simulink model "ADRClibriry"  (R2018a)
settings: Solver=VariableStepAuto  StartTime=0.0  StopTime=10.0  RelTol=1e-3
undefined symbols (not defined in the file or in its folder): sigbuilder_block
libraries: simulink x7, dspswit3 x4
(part 1 of 2)
settings Model: Creator=mengc  LastModifiedBy=mengc

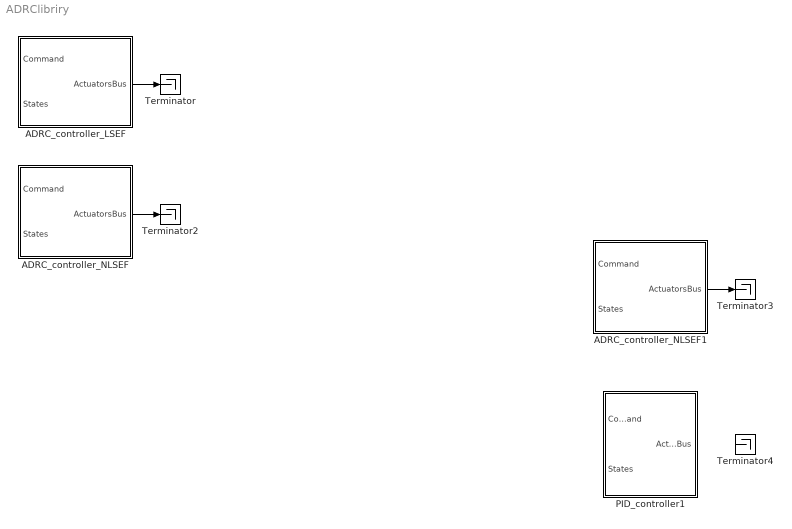
== system ADRClibriry ==
  ADRC_controller_LSEF : Subsystem
  ADRC_controller_NLSEF : Subsystem
  ADRC_controller_NLSEF1 : Subsystem
  PID_controller1 : Subsystem
  Terminator{,2..4} (4 alike) : Terminator
  wires:
  ? -> ADRC_controller_NLSEF/1(Command)  "Command"
  ADRC_controller_NLSEF/1(ActuatorsBus) -> Terminator2/1
  ? -> ADRC_controller_LSEF/1(Command)  "Command"
  ? -> ADRC_controller_LSEF/2(States)  "States"
  ? -> ADRC_controller_NLSEF/2(States)  "States"
  ADRC_controller_LSEF/1(ActuatorsBus) -> Terminator/1
  ? -> PID_controller1/1(Command)  "Command"
  ADRC_controller_NLSEF1/1(ActuatorsBus) -> Terminator3/1
  ? -> ADRC_controller_NLSEF1/2(States)  "States"
  ? -> ADRC_controller_NLSEF1/1(Command)  "Command"
  ? -> PID_controller1/2(States)  "States"

== system ADRClibriry/ADRC_controller_LSEF ==
  Command : Inport
  States : Inport  Port=2  OutDataTypeStr=Bus: StatesBus
  Bus Creator : BusCreator  Inputs=5  OutDataTypeStr=Bus: ActuatorsBus
  Bus Selector : BusSelector  OutputSignals=roll_cmd,pitch_cmd,yaw_cmd,throttle_cmd
  Bus Selector1 : BusSelector  OutputSignals=Omega_body,Euler
  Constant1 : Constant  Value=1225
  Demux : Demux  Outputs=3
  Demux1 : Demux  Outputs=3
  N-Sample Switch : dspswit3/N-Sample Switch  N=3  reset=off  TriggerType=Rising edge  Ts=0.01
      settings: SourceProductName=DSP System Toolbox  SourceProductBaseCode=DS
  Saturation : Saturate  UpperLimit=0  LowerLimit=-9.788*2
  Subsystem : Subsystem
  Subsystem2 : Subsystem
  Subsystem3 : Subsystem
  Terminator : Terminator
  Terminator1 : Terminator
  Unit Delay2 : UnitDelay  SampleTime=-1
  h_ADRC : Subsystem
  h_ADRC2 : Subsystem
  h_ADRC3 : Subsystem
  pitch_ADRC : Subsystem
  roll_ADRC : Subsystem
  yaw_ADRC : Subsystem
  ActuatorsBus : Outport  OutDataTypeStr=Bus: ActuatorsBus
  wires:
  Command/1 -> Bus Selector/1
  Unit Delay2/1 -> roll_ADRC/1(States), Bus Selector1/1, h_ADRC/1(States), yaw_ADRC/1(States), pitch_ADRC/1(States)
  yaw_ADRC/1(u_r) -> Subsystem3/3(u_r)
  Subsystem2/4(c4) -> Bus Creator/4
  Bus Selector1/2 -> Demux/1  "<Euler>"
  Bus Creator/1 -> ActuatorsBus/1  "ActuatorsBus"
  Bus Selector1/1 -> Demux1/1  "<Omega_body>"
  Demux/3 -> Terminator/1
  Subsystem3/2(u_2) -> Subsystem2/2(u_2)
  Subsystem3/1(u_1) -> Subsystem2/1(u_1)
  roll_ADRC/1("u_p ") -> Subsystem3/1(u_p)
  h_ADRC/1(a_t) -> Saturation/1
  Saturation/1 -> Subsystem/3(In3)
  Demux/1 -> Subsystem/1(In1)
  Demux/2 -> Subsystem/2(In2)
  Demux1/2 -> Subsystem3/5(q)
  Demux1/3 -> Terminator1/1
  N-Sample Switch/1 -> Bus Creator/5, Subsystem3/6(speed)  "speed"
  Constant1/1 -> N-Sample Switch/1
  Subsystem/1(speed) -> N-Sample Switch/2  "speed"
  Subsystem3/3(u_3) -> Subsystem2/3(u_3)
  Subsystem2/1(c1) -> Bus Creator/1
  Subsystem2/3(c3) -> Bus Creator/3
  Subsystem2/2(c2) -> Bus Creator/2
  pitch_ADRC/1(u_q) -> Subsystem3/2(u_q)
  Demux1/1 -> Subsystem3/4(p)
  Bus Selector/1 -> roll_ADRC/2(<roll_cmd>)  "<roll_cmd>"
  States/1 -> Unit Delay2/1
  Bus Selector/2 -> pitch_ADRC/2(<pitch_cmd>)  "<pitch_cmd>"
  Bus Selector/3 -> yaw_ADRC/2(<yaw_cmd>)  "<yaw_cmd>"
  Bus Selector/4 -> h_ADRC/2(<throttle_cmd>)  "<throttle_cmd>"

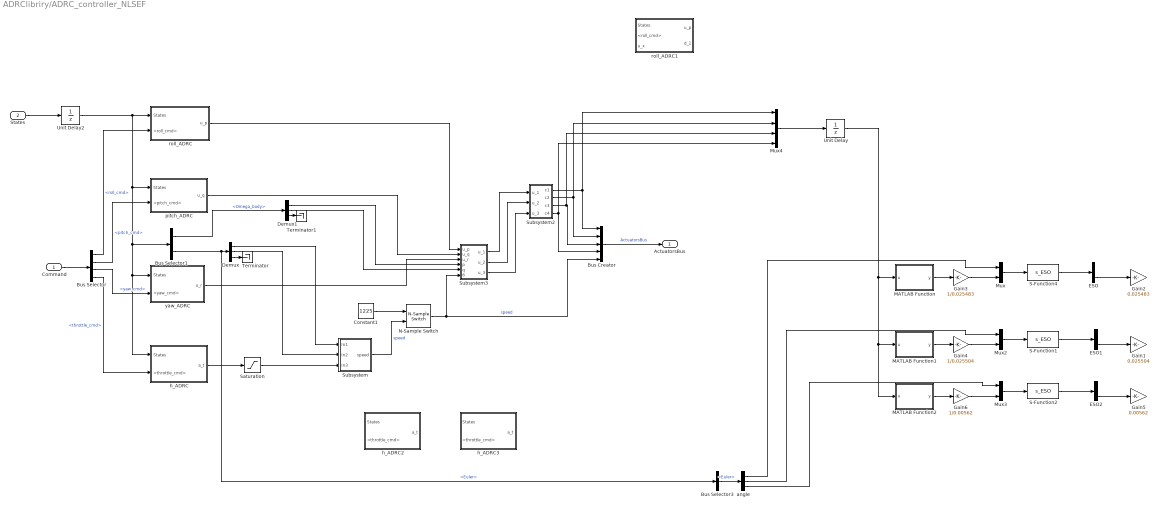
== system ADRClibriry/ADRC_controller_NLSEF ==
  Command : Inport
  States : Inport  Port=2  OutDataTypeStr=Bus: StatesBus
  Bus Creator : BusCreator  Inputs=5  OutDataTypeStr=Bus: ActuatorsBus
  Bus Selector : BusSelector  OutputSignals=roll_cmd,pitch_cmd,yaw_cmd,throttle_cmd
  Bus Selector1 : BusSelector  OutputSignals=Omega_body,Euler
  Bus Selector3 : BusSelector  OutputSignals=Euler
  Constant1 : Constant  Value=1225
  Demux : Demux  Outputs=3
  Demux1 : Demux  Outputs=3
  ESO : Demux  Outputs=3
  ESO1 : Demux  Outputs=3
  ESO2 : Demux  Outputs=3
  Gain1 : Gain  Gain=0.025504
  Gain2 : Gain  Gain=0.025483
  Gain3 : Gain  Gain=1/0.025483
  Gain4 : Gain  Gain=1/0.025504
  Gain5 : Gain  Gain=0.00562
  Gain6 : Gain  Gain=1/0.00562
  MATLAB Function : MATLAB Function  TreatAsAtomicUnit=on
  MATLAB Function1 : MATLAB Function  TreatAsAtomicUnit=on
  MATLAB Function2 : MATLAB Function  TreatAsAtomicUnit=on
  Mux : Mux  Inputs=2
  Mux2 : Mux  Inputs=2
  Mux3 : Mux  Inputs=2
  Mux4 : Mux
  N-Sample Switch : dspswit3/N-Sample Switch  N=3  reset=off  TriggerType=Rising edge  Ts=0.01
      settings: SourceProductName=DSP System Toolbox  SourceProductBaseCode=DS
  S-Function1 : S-Function  FunctionName=s_ESO  SFunctionDeploymentMode=off  EnableBusSupport=off
  S-Function2 : S-Function  FunctionName=s_ESO  SFunctionDeploymentMode=off  EnableBusSupport=off
  S-Function4 : S-Function  FunctionName=s_ESO  SFunctionDeploymentMode=off  EnableBusSupport=off
  Saturation : Saturate  UpperLimit=0  LowerLimit=-9.788*2
  Subsystem : Subsystem
  Subsystem2 : Subsystem
  Subsystem3 : Subsystem
  Terminator : Terminator
  Terminator1 : Terminator
  Unit Delay : UnitDelay  SampleTime=-1
  Unit Delay2 : UnitDelay  SampleTime=-1
  angle : Demux  Outputs=3
  h_ADRC : Subsystem
  h_ADRC2 : Subsystem
  h_ADRC3 : Subsystem
  pitch_ADRC : Subsystem
  roll_ADRC : Subsystem
  roll_ADRC1 : Subsystem
  yaw_ADRC : Subsystem
  ActuatorsBus : Outport  OutDataTypeStr=Bus: ActuatorsBus
  wires:
  Command/1 -> Bus Selector/1
  Unit Delay2/1 -> roll_ADRC/1(States), Bus Selector1/1, h_ADRC/1(States), yaw_ADRC/1(States), pitch_ADRC/1(States)
  yaw_ADRC/1(u_r) -> Subsystem3/3(u_r)
  Subsystem2/4(c4) -> Mux4/4, Bus Creator/4
  Bus Selector1/2 -> Bus Selector3/1, Demux/1  "<Euler>"
  Bus Creator/1 -> ActuatorsBus/1  "ActuatorsBus"
  Bus Selector1/1 -> Demux1/1  "<Omega_body>"
  Demux/3 -> Terminator/1
  Subsystem3/2(u_2) -> Subsystem2/2(u_2)
  Subsystem3/1(u_1) -> Subsystem2/1(u_1)
  roll_ADRC/1("u_p ") -> Subsystem3/1(u_p)
  h_ADRC/1(a_t) -> Saturation/1
  Saturation/1 -> Subsystem/3(In3)
  Demux/1 -> Subsystem/1(In1)
  Demux/2 -> Subsystem/2(In2)
  Demux1/2 -> Subsystem3/5(q)
  Demux1/3 -> Terminator1/1
  N-Sample Switch/1 -> Bus Creator/5, Subsystem3/6(speed)  "speed"
  Constant1/1 -> N-Sample Switch/1
  Subsystem/1(speed) -> N-Sample Switch/2  "speed"
  Subsystem3/3(u_3) -> Subsystem2/3(u_3)
  Subsystem2/1(c1) -> Mux4/1, Bus Creator/1
  Subsystem2/3(c3) -> Bus Creator/3, Mux4/3
  Subsystem2/2(c2) -> Mux4/2, Bus Creator/2
  pitch_ADRC/1(u_q) -> Subsystem3/2(u_q)
  Demux1/1 -> Subsystem3/4(p)
  Bus Selector/1 -> roll_ADRC/2(<roll_cmd>)  "<roll_cmd>"
  Bus Selector/2 -> pitch_ADRC/2(<pitch_cmd>)  "<pitch_cmd>"
  Bus Selector/3 -> yaw_ADRC/2(<yaw_cmd>)  "<yaw_cmd>"
  Bus Selector/4 -> h_ADRC/2(<throttle_cmd>)  "<throttle_cmd>"
  States/1 -> Unit Delay2/1
  Mux2/1 -> S-Function1/1
  MATLAB Function1/1(y) -> Gain4/1
  Gain4/1 -> Mux2/2
  S-Function2/1 -> ESO2/1
  S-Function1/1 -> ESO1/1
  MATLAB Function2/1(y) -> Gain6/1
  ESO/3 -> Gain2/1
  Mux/1 -> S-Function4/1
  Gain3/1 -> Mux/2
  MATLAB Function/1(y) -> Gain3/1
  Gain6/1 -> Mux3/2
  S-Function4/1 -> ESO/1
  ESO2/3 -> Gain5/1
  ESO1/3 -> Gain1/1
  angle/2 -> Mux2/1
  Bus Selector3/1 -> angle/1  "<Euler>"
  Mux4/1 -> Unit Delay/1
  angle/3 -> Mux3/1
  Mux3/1 -> S-Function2/1
  angle/1 -> Mux/1
  Unit Delay/1 -> MATLAB Function2/1(u), MATLAB Function1/1(u), MATLAB Function/1(u)

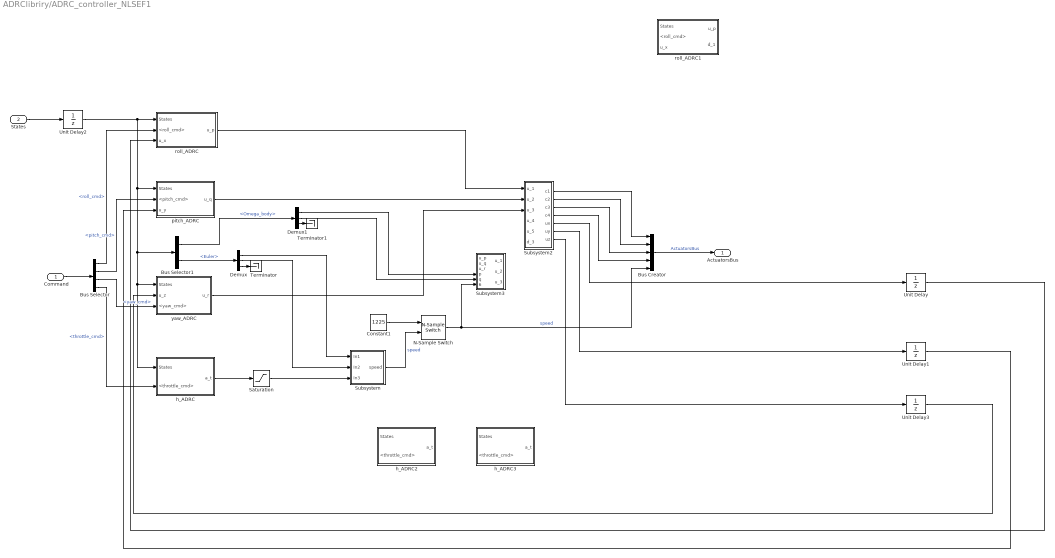
== system ADRClibriry/ADRC_controller_NLSEF1 ==
  Command : Inport
  States : Inport  Port=2  OutDataTypeStr=Bus: StatesBus
  Bus Creator : BusCreator  Inputs=5  OutDataTypeStr=Bus: ActuatorsBus
  Bus Selector : BusSelector  OutputSignals=roll_cmd,pitch_cmd,yaw_cmd,throttle_cmd
  Bus Selector1 : BusSelector  OutputSignals=Omega_body,Euler
  Constant1 : Constant  Value=1225
  Demux : Demux  Outputs=3
  Demux1 : Demux  Outputs=3
  N-Sample Switch : dspswit3/N-Sample Switch  N=3  reset=off  TriggerType=Rising edge  Ts=0.01
      settings: SourceProductName=DSP System Toolbox  SourceProductBaseCode=DS
  Saturation : Saturate  UpperLimit=0  LowerLimit=-9.788*2
  Subsystem : Subsystem
  Subsystem2 : Subsystem
  Subsystem3 : Subsystem
  Terminator : Terminator
  Terminator1 : Terminator
  Unit Delay{,1..3} (4 alike) : UnitDelay  SampleTime=-1
  h_ADRC : Subsystem
  h_ADRC2 : Subsystem
  h_ADRC3 : Subsystem
  pitch_ADRC : Subsystem
  roll_ADRC : Subsystem
  roll_ADRC1 : Subsystem
  yaw_ADRC : Subsystem
  ActuatorsBus : Outport  OutDataTypeStr=Bus: ActuatorsBus
  wires:
  Command/1 -> Bus Selector/1
  Unit Delay2/1 -> roll_ADRC/1(States), Bus Selector1/1, h_ADRC/1(States), yaw_ADRC/1(States), pitch_ADRC/1(States)
  yaw_ADRC/1(u_r) -> Subsystem2/3(u_3)
  Subsystem2/4(c4) -> Bus Creator/4
  Bus Selector1/2 -> Demux/1  "<Euler>"
  Bus Creator/1 -> ActuatorsBus/1  "ActuatorsBus"
  Bus Selector1/1 -> Demux1/1  "<Omega_body>"
  Demux/3 -> Terminator/1
  roll_ADRC/1("u_p ") -> Subsystem2/1(u_1)
  h_ADRC/1(a_t) -> Saturation/1
  Saturation/1 -> Subsystem/3(In3)
  Demux/1 -> Subsystem/1(In1)
  Demux/2 -> Subsystem/2(In2)
  Demux1/2 -> Subsystem3/5(q)
  Demux1/3 -> Terminator1/1
  N-Sample Switch/1 -> Bus Creator/5, Subsystem3/6(speed)  "speed"
  Constant1/1 -> N-Sample Switch/1
  Subsystem/1(speed) -> N-Sample Switch/2  "speed"
  Subsystem2/1(c1) -> Bus Creator/1
  Subsystem2/3(c3) -> Bus Creator/3
  Subsystem2/2(c2) -> Bus Creator/2
  pitch_ADRC/1("u_q ") -> Subsystem2/2(u_2)
  Demux1/1 -> Subsystem3/4(p)
  Bus Selector/1 -> roll_ADRC/2(<roll_cmd>)  "<roll_cmd>"
  Bus Selector/2 -> pitch_ADRC/2(<pitch_cmd>)  "<pitch_cmd>"
  Bus Selector/3 -> yaw_ADRC/3(<yaw_cmd>)  "<yaw_cmd>"
  Bus Selector/4 -> h_ADRC/2(<throttle_cmd>)  "<throttle_cmd>"
  States/1 -> Unit Delay2/1
  Unit Delay/1 -> roll_ADRC/3(u_x)
  Unit Delay3/1 -> yaw_ADRC/2(u_z)
  Unit Delay1/1 -> pitch_ADRC/3(u_y)
  Subsystem2/5(ux) -> Unit Delay/1
  Subsystem2/6(uy) -> Unit Delay1/1
  Subsystem2/7(uz) -> Unit Delay3/1

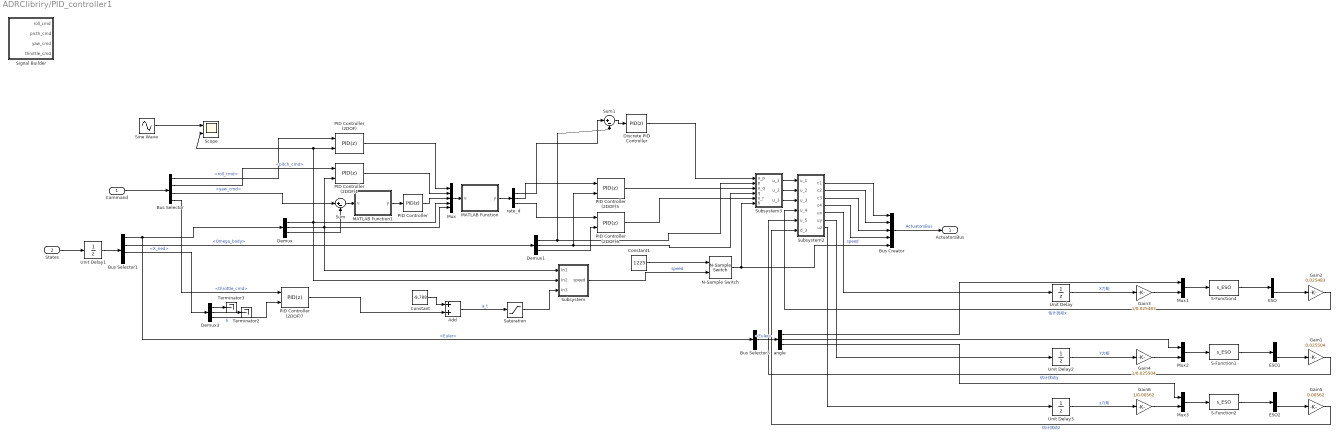
== system ADRClibriry/PID_controller1 ==
  Command : Inport
  States : Inport  Port=2  OutDataTypeStr=Bus: StatesBus
  Add : Sum
  Bus Creator : BusCreator  Inputs=5  OutDataTypeStr=Bus: ActuatorsBus
  Bus Selector : BusSelector  OutputSignals=roll_cmd,pitch_cmd,yaw_cmd,throttle_cmd
  Bus Selector1 : BusSelector  OutputSignals=Euler,Omega_body,X_ned,V_ned
  Bus Selector3 : BusSelector  OutputSignals=Euler
  Constant : Constant  Value=-9.788
  Constant1 : Constant  Value=1225
  Demux : Demux  Outputs=3
  Demux1 : Demux  Outputs=3
  Demux3 : Demux  Outputs=3
  Discrete PID Controller : simulink/Continuous/PID Controller  Controller=PID  TimeDomain=Discrete-time  SampleTime=-1  IntegratorMethod=Forward Euler  FilterMethod=Forward Euler  Form=Parallel  UseFilter=on  ControllerParametersSource=internal  P=0.4  I=0.08  D=0  N=100  InitialConditionSource=internal  InitialConditionForIntegrator=0  InitialConditionForFilter=0  ExternalReset=none  LimitOutput=off  UpperSaturationLimit=inf  LowerSaturationLimit=-inf  LinearizeAsGain=off  AntiWindupMode=none  Kb=1  TrackingMode=off  Kt=1  PParamMin=[]  PParamMax=[]  IParamMin=[]  IParamMax=[]  DParamMin=[]  DParamMax=[]  NParamMin=[]  NParamMax=[]  KbParamMin=[]  KbParamMax=[]  KtParamMin=[]  KtParamMax=[]  POutMin=[]  POutMax=[]  IOutMin=[]  IOutMax=[]  DOutMin=[]  DOutMax=[]  NOutMin=[]  NOutMax=[]  KbOutMin=[]  KbOutMax=[]  KtOutMin=[]  KtOutMax=[]  IntegratorOutMin=[]  IntegratorOutMax=[]  FilterOutMin=[]  FilterOutMax=[]  SumOutMin=[]  SumOutMax=[]  SumI1OutMin=[]  SumI1OutMax=[]  SumI2OutMin=[]  SumI2OutMax=[]  SumI3OutMin=[]  SumI3OutMax=[]  SumDOutMin=[]  SumDOutMax=[]  SaturationOutMin=[]  SaturationOutMax=[]  IntegratorContinuousStateAttributes=''  IntegratorStateMustResolveToSignalObject=off  IntegratorRTWStateStorageClass=Auto  FilterContinuousStateAttributes=''  FilterStateMustResolveToSignalObject=off  FilterRTWStateStorageClass=Auto  DifferentiatorICPrevScaledInput=0  DifferentiatorOutMin=[]  DifferentiatorOutMax=[]  FilterDiffOutCoefMin=[]  FilterDiffOutCoefMax=[]  SumDenOutMin=[]  SumDenOutMax=[]  SumNumOutMin=[]  SumNumOutMax=[]  ReciprocalOutMin=[]  ReciprocalOutMax=[]  DivideOutMin=[]  DivideOutMax=[]  TunerSelectOption=Transfer Function Based (PID Tuner App)
  ESO : Demux  Outputs=3
  ESO1 : Demux  Outputs=3
  ESO2 : Demux  Outputs=3
  Gain1 : Gain  Gain=0.025504
  Gain2 : Gain  Gain=0.025483
  Gain3 : Gain  Gain=1/0.025483
  Gain4 : Gain  Gain=1/0.025504
  Gain5 : Gain  Gain=0.00562
  Gain6 : Gain  Gain=1/0.00562
  MATLAB Function : MATLAB Function  TreatAsAtomicUnit=on
  MATLAB Function1 : MATLAB Function  TreatAsAtomicUnit=on
  Mux : Mux  Inputs=5
  Mux1 : Mux  Inputs=2
  Mux2 : Mux  Inputs=2
  Mux3 : Mux  Inputs=2
  N-Sample Switch : dspswit3/N-Sample Switch  N=3  reset=off  TriggerType=Rising edge  Ts=0.01
      settings: SourceProductName=DSP System Toolbox  SourceProductBaseCode=DS
  PID Controller : simulink/Continuous/PID Controller  Controller=PID  TimeDomain=Discrete-time  SampleTime=-1  IntegratorMethod=Forward Euler  FilterMethod=Forward Euler  Form=Parallel  UseFilter=on  ControllerParametersSource=internal  P=5  I=0.8  D=0  N=100  InitialConditionSource=internal  InitialConditionForIntegrator=0  InitialConditionForFilter=0  ExternalReset=none  LimitOutput=off  UpperSaturationLimit=inf  LowerSaturationLimit=-inf  LinearizeAsGain=on  AntiWindupMode=none  Kb=1  TrackingMode=off  Kt=1  PParamMin=[]  PParamMax=[]  IParamMin=[]  IParamMax=[]  DParamMin=[]  DParamMax=[]  NParamMin=[]  NParamMax=[]  KbParamMin=[]  KbParamMax=[]  KtParamMin=[]  KtParamMax=[]  POutMin=[]  POutMax=[]  IOutMin=[]  IOutMax=[]  DOutMin=[]  DOutMax=[]  NOutMin=[]  NOutMax=[]  KbOutMin=[]  KbOutMax=[]  KtOutMin=[]  KtOutMax=[]  IntegratorOutMin=[]  IntegratorOutMax=[]  FilterOutMin=[]  FilterOutMax=[]  SumOutMin=[]  SumOutMax=[]  SumI1OutMin=[]  SumI1OutMax=[]  SumI2OutMin=[]  SumI2OutMax=[]  SumI3OutMin=[]  SumI3OutMax=[]  SumDOutMin=[]  SumDOutMax=[]  SaturationOutMin=[]  SaturationOutMax=[]  IntegratorContinuousStateAttributes=''  IntegratorStateMustResolveToSignalObject=off  IntegratorRTWStateStorageClass=Auto  FilterContinuousStateAttributes=''  FilterStateMustResolveToSignalObject=off  FilterRTWStateStorageClass=Auto  DifferentiatorICPrevScaledInput=0  DifferentiatorOutMin=[]  DifferentiatorOutMax=[]  FilterDiffOutCoefMin=[]  FilterDiffOutCoefMax=[]  SumDenOutMin=[]  SumDenOutMax=[]  SumNumOutMin=[]  SumNumOutMax=[]  ReciprocalOutMin=[]  ReciprocalOutMax=[]  DivideOutMin=[]  DivideOutMax=[]  TunerSelectOption=Transfer Function Based (PID Tuner App)
  PID Controller (2DOF) : simulink/Continuous/PID Controller (2DOF)  Controller=PID  TimeDomain=Discrete-time  SampleTime=-1  IntegratorMethod=Forward Euler  FilterMethod=Forward Euler  Form=Parallel  UseFilter=on  ControllerParametersSource=internal  P=7  I=2  D=0  N=100  b=1  c=1  InitialConditionSource=internal  InitialConditionForIntegrator=0  InitialConditionForFilter=0  ExternalReset=none  LimitOutput=off  UpperSaturationLimit=inf  LowerSaturationLimit=-inf  LinearizeAsGain=on  AntiWindupMode=none  Kb=1  TrackingMode=off  Kt=1  PParamMin=[]  PParamMax=[]  IParamMin=[]  IParamMax=[]  DParamMin=[]  DParamMax=[]  NParamMin=[]  NParamMax=[]  bParamMin=[]  bParamMax=[]  cParamMin=[]  cParamMax=[]  KbParamMin=[]  KbParamMax=[]  KtParamMin=[]  KtParamMax=[]  POutMin=[]  POutMax=[]  IOutMin=[]  IOutMax=[]  DOutMin=[]  DOutMax=[]  NOutMin=[]  NOutMax=[]  bOutMin=[]  bOutMax=[]  cOutMin=[]  cOutMax=[]  KbOutMin=[]  KbOutMax=[]  KtOutMin=[]  KtOutMax=[]  IntegratorOutMin=[]  IntegratorOutMax=[]  FilterOutMin=[]  FilterOutMax=[]  SumOutMin=[]  SumOutMax=[]  Sum1OutMin=[]  Sum1OutMax=[]  Sum2OutMin=[]  Sum2OutMax=[]  Sum3OutMin=[]  Sum3OutMax=[]  SumI1OutMin=[]  SumI1OutMax=[]  SumI2OutMin=[]  SumI2OutMax=[]  SumI3OutMin=[]  SumI3OutMax=[]  SumDOutMin=[]  SumDOutMax=[]  SaturationOutMin=[]  SaturationOutMax=[]  IntegratorContinuousStateAttributes=''  IntegratorStateMustResolveToSignalObject=off  IntegratorRTWStateStorageClass=Auto  FilterContinuousStateAttributes=''  FilterStateMustResolveToSignalObject=off  FilterRTWStateStorageClass=Auto  DifferentiatorICPrevScaledInput=0  DifferentiatorOutMin=[]  DifferentiatorOutMax=[]  FilterDiffOutCoefMin=[]  FilterDiffOutCoefMax=[]  SumDenOutMin=[]  SumDenOutMax=[]  SumNumOutMin=[]  SumNumOutMax=[]  ReciprocalOutMin=[]  ReciprocalOutMax=[]  DivideOutMin=[]  DivideOutMax=[]  TunerSelectOption=Transfer Function Based (PID Tuner App)
  PID Controller (2DOF)1 : simulink/Continuous/PID Controller (2DOF)  Controller=PID  TimeDomain=Discrete-time  SampleTime=-1  IntegratorMethod=Forward Euler  FilterMethod=Forward Euler  Form=Parallel  UseFilter=on  ControllerParametersSource=internal  P=7  I=2  D=0  N=100  b=1  c=1  InitialConditionSource=internal  InitialConditionForIntegrator=0  InitialConditionForFilter=0  ExternalReset=none  LimitOutput=off  UpperSaturationLimit=inf  LowerSaturationLimit=-inf  LinearizeAsGain=on  AntiWindupMode=none  Kb=1  TrackingMode=off  Kt=1  PParamMin=[]  PParamMax=[]  IParamMin=[]  IParamMax=[]  DParamMin=[]  DParamMax=[]  NParamMin=[]  NParamMax=[]  bParamMin=[]  bParamMax=[]  cParamMin=[]  cParamMax=[]  KbParamMin=[]  KbParamMax=[]  KtParamMin=[]  KtParamMax=[]  POutMin=[]  POutMax=[]  IOutMin=[]  IOutMax=[]  DOutMin=[]  DOutMax=[]  NOutMin=[]  NOutMax=[]  bOutMin=[]  bOutMax=[]  cOutMin=[]  cOutMax=[]  KbOutMin=[]  KbOutMax=[]  KtOutMin=[]  KtOutMax=[]  IntegratorOutMin=[]  IntegratorOutMax=[]  FilterOutMin=[]  FilterOutMax=[]  SumOutMin=[]  SumOutMax=[]  Sum1OutMin=[]  Sum1OutMax=[]  Sum2OutMin=[]  Sum2OutMax=[]  Sum3OutMin=[]  Sum3OutMax=[]  SumI1OutMin=[]  SumI1OutMax=[]  SumI2OutMin=[]  SumI2OutMax=[]  SumI3OutMin=[]  SumI3OutMax=[]  SumDOutMin=[]  SumDOutMax=[]  SaturationOutMin=[]  SaturationOutMax=[]  IntegratorContinuousStateAttributes=''  IntegratorStateMustResolveToSignalObject=off  IntegratorRTWStateStorageClass=Auto  FilterContinuousStateAttributes=''  FilterStateMustResolveToSignalObject=off  FilterRTWStateStorageClass=Auto  DifferentiatorICPrevScaledInput=0  DifferentiatorOutMin=[]  DifferentiatorOutMax=[]  FilterDiffOutCoefMin=[]  FilterDiffOutCoefMax=[]  SumDenOutMin=[]  SumDenOutMax=[]  SumNumOutMin=[]  SumNumOutMax=[]  ReciprocalOutMin=[]  ReciprocalOutMax=[]  DivideOutMin=[]  DivideOutMax=[]  TunerSelectOption=Transfer Function Based (PID Tuner App)
  PID Controller (2DOF)5 : simulink/Continuous/PID Controller (2DOF)  Controller=PID  TimeDomain=Discrete-time  SampleTime=-1  IntegratorMethod=Forward Euler  FilterMethod=Forward Euler  Form=Parallel  UseFilter=on  ControllerParametersSource=internal  P=0.4  I=0.08  D=0  N=100  b=1  c=1  InitialConditionSource=internal  InitialConditionForIntegrator=0  InitialConditionForFilter=0  ExternalReset=none  LimitOutput=off  UpperSaturationLimit=inf  LowerSaturationLimit=-inf  LinearizeAsGain=on  AntiWindupMode=none  Kb=1  TrackingMode=off  Kt=1  PParamMin=[]  PParamMax=[]  IParamMin=[]  IParamMax=[]  DParamMin=[]  DParamMax=[]  NParamMin=[]  NParamMax=[]  bParamMin=[]  bParamMax=[]  cParamMin=[]  cParamMax=[]  KbParamMin=[]  KbParamMax=[]  KtParamMin=[]  KtParamMax=[]  POutMin=[]  POutMax=[]  IOutMin=[]  IOutMax=[]  DOutMin=[]  DOutMax=[]  NOutMin=[]  NOutMax=[]  bOutMin=[]  bOutMax=[]  cOutMin=[]  cOutMax=[]  KbOutMin=[]  KbOutMax=[]  KtOutMin=[]  KtOutMax=[]  IntegratorOutMin=[]  IntegratorOutMax=[]  FilterOutMin=[]  FilterOutMax=[]  SumOutMin=[]  SumOutMax=[]  Sum1OutMin=[]  Sum1OutMax=[]  Sum2OutMin=[]  Sum2OutMax=[]  Sum3OutMin=[]  Sum3OutMax=[]  SumI1OutMin=[]  SumI1OutMax=[]  SumI2OutMin=[]  SumI2OutMax=[]  SumI3OutMin=[]  SumI3OutMax=[]  SumDOutMin=[]  SumDOutMax=[]  SaturationOutMin=[]  SaturationOutMax=[]  IntegratorContinuousStateAttributes=''  IntegratorStateMustResolveToSignalObject=off  IntegratorRTWStateStorageClass=Auto  FilterContinuousStateAttributes=''  FilterStateMustResolveToSignalObject=off  FilterRTWStateStorageClass=Auto  DifferentiatorICPrevScaledInput=0  DifferentiatorOutMin=[]  DifferentiatorOutMax=[]  FilterDiffOutCoefMin=[]  FilterDiffOutCoefMax=[]  SumDenOutMin=[]  SumDenOutMax=[]  SumNumOutMin=[]  SumNumOutMax=[]  ReciprocalOutMin=[]  ReciprocalOutMax=[]  DivideOutMin=[]  DivideOutMax=[]  TunerSelectOption=Transfer Function Based (PID Tuner App)
  PID Controller (2DOF)6 : simulink/Continuous/PID Controller (2DOF)  Controller=PID  TimeDomain=Discrete-time  SampleTime=-1  IntegratorMethod=Forward Euler  FilterMethod=Forward Euler  Form=Parallel  UseFilter=on  ControllerParametersSource=internal  P=0.3  I=0.05  D=0  N=100  b=1  c=1  InitialConditionSource=internal  InitialConditionForIntegrator=0  InitialConditionForFilter=0  ExternalReset=none  LimitOutput=off  UpperSaturationLimit=inf  LowerSaturationLimit=-inf  LinearizeAsGain=on  AntiWindupMode=none  Kb=1  TrackingMode=off  Kt=1  PParamMin=[]  PParamMax=[]  IParamMin=[]  IParamMax=[]  DParamMin=[]  DParamMax=[]  NParamMin=[]  NParamMax=[]  bParamMin=[]  bParamMax=[]  cParamMin=[]  cParamMax=[]  KbParamMin=[]  KbParamMax=[]  KtParamMin=[]  KtParamMax=[]  POutMin=[]  POutMax=[]  IOutMin=[]  IOutMax=[]  DOutMin=[]  DOutMax=[]  NOutMin=[]  NOutMax=[]  bOutMin=[]  bOutMax=[]  cOutMin=[]  cOutMax=[]  KbOutMin=[]  KbOutMax=[]  KtOutMin=[]  KtOutMax=[]  IntegratorOutMin=[]  IntegratorOutMax=[]  FilterOutMin=[]  FilterOutMax=[]  SumOutMin=[]  SumOutMax=[]  Sum1OutMin=[]  Sum1OutMax=[]  Sum2OutMin=[]  Sum2OutMax=[]  Sum3OutMin=[]  Sum3OutMax=[]  SumI1OutMin=[]  SumI1OutMax=[]  SumI2OutMin=[]  SumI2OutMax=[]  SumI3OutMin=[]  SumI3OutMax=[]  SumDOutMin=[]  SumDOutMax=[]  SaturationOutMin=[]  SaturationOutMax=[]  IntegratorContinuousStateAttributes=''  IntegratorStateMustResolveToSignalObject=off  IntegratorRTWStateStorageClass=Auto  FilterContinuousStateAttributes=''  FilterStateMustResolveToSignalObject=off  FilterRTWStateStorageClass=Auto  DifferentiatorICPrevScaledInput=0  DifferentiatorOutMin=[]  DifferentiatorOutMax=[]  FilterDiffOutCoefMin=[]  FilterDiffOutCoefMax=[]  SumDenOutMin=[]  SumDenOutMax=[]  SumNumOutMin=[]  SumNumOutMax=[]  ReciprocalOutMin=[]  ReciprocalOutMax=[]  DivideOutMin=[]  DivideOutMax=[]  TunerSelectOption=Transfer Function Based (PID Tuner App)
  PID Controller (2DOF)7 : simulink/Continuous/PID Controller (2DOF)  Controller=PID  TimeDomain=Discrete-time  SampleTime=-1  IntegratorMethod=Forward Euler  FilterMethod=Forward Euler  Form=Parallel  UseFilter=on  ControllerParametersSource=internal  P=2.3  I=0.2  D=2.3  N=100  b=1  c=1  InitialConditionSource=internal  InitialConditionForIntegrator=0  InitialConditionForFilter=0  ExternalReset=none  LimitOutput=off  UpperSaturationLimit=inf  LowerSaturationLimit=-inf  LinearizeAsGain=on  AntiWindupMode=none  Kb=1  TrackingMode=off  Kt=1  PParamMin=[]  PParamMax=[]  IParamMin=[]  IParamMax=[]  DParamMin=[]  DParamMax=[]  NParamMin=[]  NParamMax=[]  bParamMin=[]  bParamMax=[]  cParamMin=[]  cParamMax=[]  KbParamMin=[]  KbParamMax=[]  KtParamMin=[]  KtParamMax=[]  POutMin=[]  POutMax=[]  IOutMin=[]  IOutMax=[]  DOutMin=[]  DOutMax=[]  NOutMin=[]  NOutMax=[]  bOutMin=[]  bOutMax=[]  cOutMin=[]  cOutMax=[]  KbOutMin=[]  KbOutMax=[]  KtOutMin=[]  KtOutMax=[]  IntegratorOutMin=[]  IntegratorOutMax=[]  FilterOutMin=[]  FilterOutMax=[]  SumOutMin=[]  SumOutMax=[]  Sum1OutMin=[]  Sum1OutMax=[]  Sum2OutMin=[]  Sum2OutMax=[]  Sum3OutMin=[]  Sum3OutMax=[]  SumI1OutMin=[]  SumI1OutMax=[]  SumI2OutMin=[]  SumI2OutMax=[]  SumI3OutMin=[]  SumI3OutMax=[]  SumDOutMin=[]  SumDOutMax=[]  SaturationOutMin=[]  SaturationOutMax=[]  IntegratorContinuousStateAttributes=''  IntegratorStateMustResolveToSignalObject=off  IntegratorRTWStateStorageClass=Auto  FilterContinuousStateAttributes=''  FilterStateMustResolveToSignalObject=off  FilterRTWStateStorageClass=Auto  DifferentiatorICPrevScaledInput=0  DifferentiatorOutMin=[]  DifferentiatorOutMax=[]  FilterDiffOutCoefMin=[]  FilterDiffOutCoefMax=[]  SumDenOutMin=[]  SumDenOutMax=[]  SumNumOutMin=[]  SumNumOutMax=[]  ReciprocalOutMin=[]  ReciprocalOutMax=[]  DivideOutMin=[]  DivideOutMax=[]  TunerSelectOption=Transfer Function Based (PID Tuner App)
  S-Function1 : S-Function  FunctionName=s_ESO  SFunctionDeploymentMode=off  EnableBusSupport=off
  S-Function2 : S-Function  FunctionName=s_ESO  SFunctionDeploymentMode=off  EnableBusSupport=off
  S-Function4 : S-Function  FunctionName=s_ESO  SFunctionDeploymentMode=off  EnableBusSupport=off
  Saturation : Saturate  UpperLimit=0  LowerLimit=-2*9.788
  Scope : Scope  NumInputPorts=2
  Signal Builder : Subsystem  Tag=STV Subsys  LoadFcn=sigbuilder_block('load');  StartFcn=sigbuilder_block('start');  StopFcn=sigbuilder_block('stop');  ClipboardFcn=sigbuilder_block('clipboard');  mask(Sigbuilder block){tuvar=[0:10]}
      mask help: Simulink:masks:SigbuilderBlock_MD
      mask init:
      | if ~strcmp(get_param(bdroot(gcbh),'SimulationStatus'),'stopped') tuvar = sigbuilder_block('maskInit'); end
      settings: CopyFcn=sigbuilder_block('copy');  DeleteFcn=sigbuilder_block('delete');  ModelCloseFcn=sigbuilder_block('modelClose');  PreSaveFcn=sigbuilder_block('preSave');  PauseFcn=sigbuilder_block('pause');  ContinueFcn=sigbuilder_block('continue');  NameChangeFcn=sigbuilder_block('namechange');  OpenFcn=sigbuilder_block('open',[5.5 30 949 419 ]);  CloseFcn=sigbuilder_block('close');
      mask Display: plot(0, 0, 100, 100,[2, 2, 32, 32, 2], [68, 8, 8, 68, 68],[32, 2], [38, 38], [32, 19, 2],[53, 60, 44], [32, 17, 17, 2],[16, 16, 31, 31]);txt = getActiveGroup(gcbh);text(2, 100, txt,'verticalAlignment', 'top');
  Sine Wave : Sin  Amplitude=0.2  Frequency=2*pi*1  SampleTime=0.01
  Subsystem : Subsystem
  Subsystem2 : Subsystem
  Subsystem3 : Subsystem
  Sum : Sum  Inputs=|+-
  Sum1 : Sum  Inputs=|+-
  Terminator2 : Terminator
  Terminator3 : Terminator
  Unit Delay{,1..3} (4 alike) : UnitDelay  SampleTime=-1
  angle : Demux  Outputs=3
  rate_d : Demux  Outputs=3
  ActuatorsBus : Outport  OutDataTypeStr=Bus: ActuatorsBus
  wires:
  PID Controller/1 -> Mux/3
  Bus Selector/3 -> Sum/1  "<yaw_cmd>"
  Demux/3 -> Sum/2
  Bus Selector1/3 -> Demux3/1  "<X_ned>"
  PID Controller (2DOF)6/1 -> Subsystem3/5(u_r)
  PID Controller (2DOF)7/1 -> Add/2
  Demux1/1 -> Sum1/2, Subsystem3/2(p)
  Bus Selector/2 -> PID Controller (2DOF)1/1  "<pitch_cmd>"
  Bus Selector1/2 -> Demux1/1  "<Omega_body>"
  Bus Selector1/1 -> Demux/1, Bus Selector3/1  "<Euler>"
  Sum/1 -> MATLAB Function1/1(u)
  PID Controller (2DOF)/1 -> Mux/1
  Demux3/2 -> Terminator2/1
  Demux/2 -> PID Controller (2DOF)1/2, Mux/5, Subsystem/1(In1)
  Demux1/2 -> Subsystem3/4(q), PID Controller (2DOF)5/2
  rate_d/3 -> PID Controller (2DOF)6/1
  PID Controller (2DOF)1/1 -> Mux/2
  Demux/1 -> Subsystem/2(In2), Mux/4, Scope/2, PID Controller (2DOF)/2
  Demux1/3 -> PID Controller (2DOF)6/2
  MATLAB Function1/1(y) -> PID Controller/1
  PID Controller (2DOF)5/1 -> Subsystem3/3(u_q)
  Demux3/1 -> Terminator3/1
  rate_d/2 -> PID Controller (2DOF)5/1
  Bus Selector/4 -> PID Controller (2DOF)7/1  "<throttle_cmd>"
  rate_d/1 -> Sum1/1
  Mux/1 -> MATLAB Function/1(u)
  Command/1 -> Bus Selector/1
  Bus Creator/1 -> ActuatorsBus/1  "ActuatorsBus"
  Constant1/1 -> N-Sample Switch/1
  Subsystem/1(speed) -> N-Sample Switch/2  "speed"
  N-Sample Switch/1 -> Bus Creator/5, Subsystem3/6(speed)  "speed"
  Demux3/3 -> PID Controller (2DOF)7/2  "h"
  MATLAB Function/1(y) -> rate_d/1
  Discrete PID Controller/1 -> Subsystem3/1(u_p)
  States/1 -> Unit Delay1/1
  Unit Delay1/1 -> Bus Selector1/1
  Saturation/1 -> Subsystem/3(In3)
  Add/1 -> Saturation/1  "a_t"
  Constant/1 -> Add/1
  Sum1/1 -> Discrete PID Controller/1
  Sine Wave/1 -> Scope/1
  Bus Selector/1 -> PID Controller (2DOF)/1  "<roll_cmd>"
  Unit Delay/1 -> Gain3/1  "X力矩"
  angle/1 -> Mux1/1
  S-Function4/1 -> ESO/1
  Gain3/1 -> Mux1/2
  Mux3/1 -> S-Function2/1
  Subsystem2/4(c4) -> Bus Creator/4
  Mux1/1 -> S-Function4/1
  angle/2 -> Mux2/1
  ESO/3 -> Gain2/1
  ESO1/3 -> Gain1/1
  S-Function2/1 -> ESO2/1
  Gain6/1 -> Mux3/2
  Gain4/1 -> Mux2/2
  Mux2/1 -> S-Function1/1
  Subsystem2/2(c2) -> Bus Creator/2
  S-Function1/1 -> ESO1/1
  Unit Delay3/1 -> Gain6/1  "z力矩"
  angle/3 -> Mux3/1
  Subsystem2/1(c1) -> Bus Creator/1
  Unit Delay2/1 -> Gain4/1  "Y力矩"
  Bus Selector3/1 -> angle/1  "<Euler>"
  Subsystem2/3(c3) -> Bus Creator/3
  ESO2/3 -> Gain5/1
  Subsystem3/1(u_1) -> Subsystem2/1(u_1)
  Subsystem3/2(u_2) -> Subsystem2/2(u_2)
  Subsystem3/3(u_3) -> Subsystem2/3(u_3)
  Subsystem2/5(ux) -> Unit Delay/1
  Subsystem2/6(uy) -> Unit Delay2/1
  Subsystem2/7(uz) -> Unit Delay3/1
  Gain2/1 -> Subsystem2/4(u_4)  "估计扰动x"
  Gain1/1 -> Subsystem2/5(u_5)  "估计扰动y"
  Gain5/1 -> Subsystem2/6(d_3)  "估计扰动z"

== system ADRClibriry/ADRC_controller_LSEF/Subsystem ==
  In1 : Inport
  In2 : Inport  Port=2
  In3 : Inport  Port=3
  Divide : Product  Inputs=*/
  Gain : Gain  Gain=-1225^2/9.788
  Product : Product
  Saturation1 : Saturate  UpperLimit=1  LowerLimit=0.5
  Sqrt : Sqrt  SaturateOnIntegerOverflow=on
  Trigonometric Function : Trigonometry  Operator=cos
  Trigonometric Function1 : Trigonometry  Operator=cos
  speed : Outport
  wires:
  Saturation1/1 -> Divide/2
  Trigonometric Function/1 -> Product/1
  In3/1 -> Divide/1
  Trigonometric Function1/1 -> Product/2
  In2/1 -> Trigonometric Function/1
  Product/1 -> Saturation1/1
  In1/1 -> Trigonometric Function1/1
  Divide/1 -> Gain/1
  Gain/1 -> Sqrt/1
  Sqrt/1 -> speed/1

== system ADRClibriry/ADRC_controller_LSEF/Subsystem2 ==
  u_1 : Inport
  u_2 : Inport  Port=2
  u_3 : Inport  Port=3
  Demux3 : Demux
  MATLAB Function : MATLAB Function  TreatAsAtomicUnit=on
  Mux : Mux  Inputs=3
  Saturation{1..4} (4 alike) : Saturate  UpperLimit=0.3491  LowerLimit=-0.3491
  c1 : Outport
  c2 : Outport  Port=2
  c3 : Outport  Port=3
  c4 : Outport  Port=4
  wires:
  Mux/1 -> MATLAB Function/1(u)
  Demux3/4 -> Saturation4/1
  Saturation3/1 -> c3/1  "c3"
  u_3/1 -> Mux/3
  u_1/1 -> Mux/1
  Saturation1/1 -> c1/1  "c1"
  Demux3/1 -> Saturation1/1
  Saturation4/1 -> c4/1  "c4"
  Demux3/2 -> Saturation2/1
  MATLAB Function/1(y) -> Demux3/1
  u_2/1 -> Mux/2
  Saturation2/1 -> c2/1  "c2"
  Demux3/3 -> Saturation3/1

== system ADRClibriry/ADRC_controller_LSEF/Subsystem3 ==
  u_p : Inport
  u_q : Inport  Port=2
  u_r : Inport  Port=3
  p : Inport  Port=4
  q : Inport  Port=5
  speed : Inport  Port=6
  Add1 : Sum
  Add2 : Sum  Inputs=+-
  Add3 : Sum  Inputs=+-
  Constant1 : Constant  Value=0.000029
  Constant2 : Constant  Value=0.04238
  Product{,1..3} (4 alike) : Product
  u_1 : Outport
  u_2 : Outport  Port=2
  u_3 : Outport  Port=3
  wires:
  Add3/1 -> u_3/1
  Add1/1 -> u_1/1
  Constant1/1 -> Product1/1, Product/2
  q/1 -> Product/1
  Product1/1 -> Product2/1
  Constant2/1 -> Add3/2
  u_p/1 -> Add1/2
  p/1 -> Product1/2
  Add2/1 -> u_2/1
  Product3/1 -> Add1/1
  speed/1 -> Product3/2, Product2/2
  Product/1 -> Product3/1
  Product2/1 -> Add2/2
  u_q/1 -> Add2/1
  u_r/1 -> Add3/1

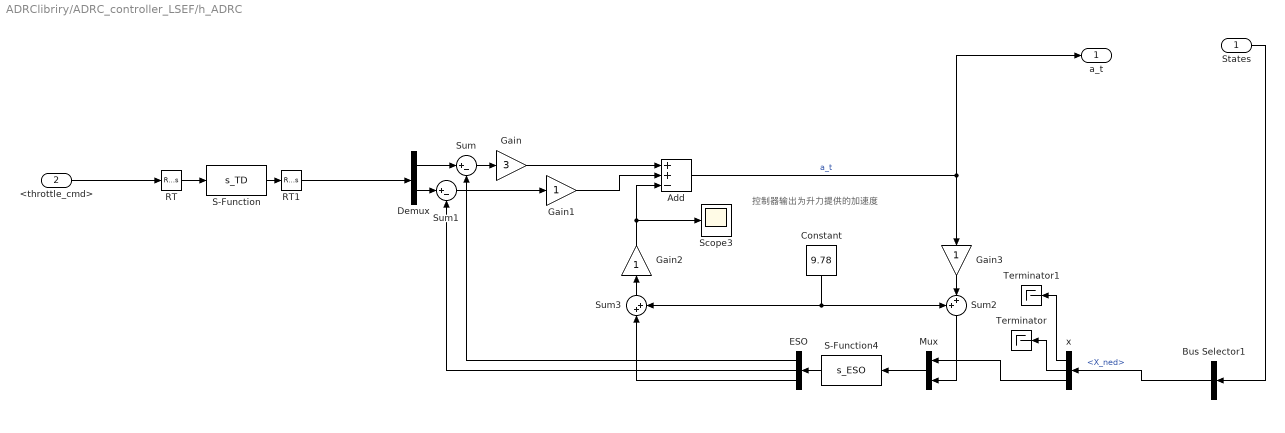
== system ADRClibriry/ADRC_controller_LSEF/h_ADRC ==
  note: 控制器输出为升力提供的加速度
  States : Inport  OutDataTypeStr=Bus: StatesBus
  <throttle_cmd> : Inport  Port=2
  Add : Sum  Inputs=++-
  Bus Selector1 : BusSelector  OutputSignals=X_ned
  Constant : Constant  Value=9.78
  Demux : Demux  Outputs=2
  ESO : Demux  Outputs=3
  Gain : Gain  Gain=3
  Gain1 : Gain
  Gain2 : Gain
  Gain3 : Gain
  Mux : Mux  Inputs=2
  RT : RateTransition  OutPortSampleTime=0.05
  RT1 : RateTransition  OutPortSampleTime=0.01
  S-Function : S-Function  FunctionName=s_TD  SFunctionDeploymentMode=off  EnableBusSupport=off
  S-Function4 : S-Function  FunctionName=s_ESO  SFunctionDeploymentMode=off  EnableBusSupport=off
  Scope3 : Scope
  Sum : Sum  Inputs=|+-
  Sum1 : Sum  Inputs=|+-
  Sum2 : Sum  Inputs=++|
  Sum3 : Sum  Inputs=|++
  Terminator : Terminator
  Terminator1 : Terminator
  x : Demux  Outputs=3
  a_t : Outport
  wires:
  Gain1/1 -> Add/2
  Mux/1 -> S-Function4/1
  States/1 -> Bus Selector1/1
  ESO/1 -> Sum/2
  Gain3/1 -> Sum2/2
  ESO/3 -> Sum3/1
  <throttle_cmd>/1 -> RT/1
  ESO/2 -> Sum1/2
  Bus Selector1/1 -> x/1  "<X_ned>"
  RT/1 -> S-Function/1
  S-Function4/1 -> ESO/1
  Sum1/1 -> Gain1/1
  Gain/1 -> Add/1
  RT1/1 -> Demux/1
  Demux/2 -> Sum1/1
  Gain2/1 -> Add/3, Scope3/1
  S-Function/1 -> RT1/1
  Sum/1 -> Gain/1
  Demux/1 -> Sum/1
  x/3 -> Mux/1
  x/2 -> Terminator/1
  x/1 -> Terminator1/1
  Add/1 -> a_t/1, Gain3/1  "a_t"
  Sum2/1 -> Mux/2
  Sum3/1 -> Gain2/1
  Constant/1 -> Sum3/2, Sum2/1

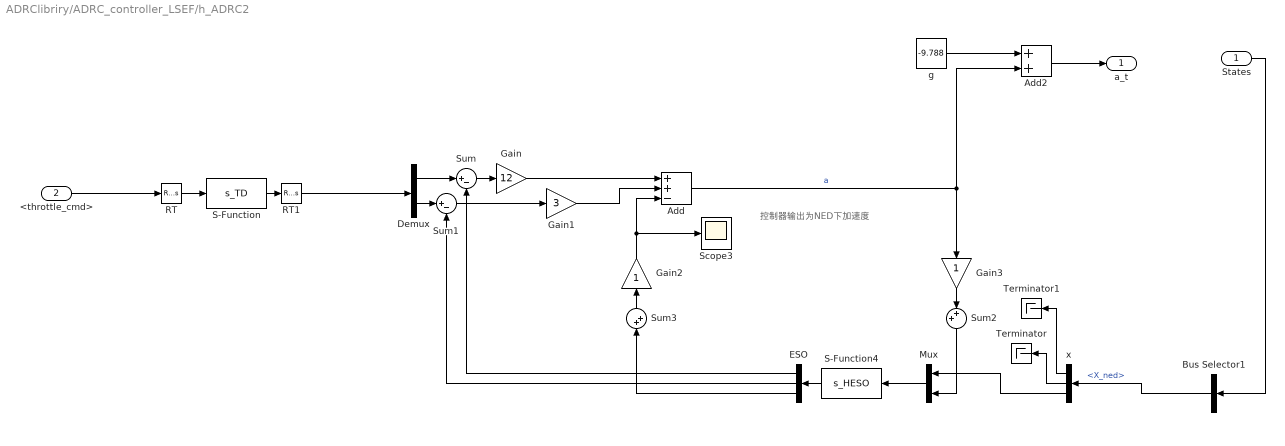
== system ADRClibriry/ADRC_controller_LSEF/h_ADRC2 ==
  note: 控制器输出为NED下加速度
  States : Inport  OutDataTypeStr=Bus: StatesBus
  <throttle_cmd> : Inport  Port=2
  Add : Sum  Inputs=++-
  Add2 : Sum
  Bus Selector1 : BusSelector  OutputSignals=X_ned
  Demux : Demux  Outputs=2
  ESO : Demux  Outputs=3
  Gain : Gain  Gain=12
  Gain1 : Gain  Gain=3
  Gain2 : Gain
  Gain3 : Gain
  Mux : Mux  Inputs=2
  RT : RateTransition  OutPortSampleTime=0.05
  RT1 : RateTransition  OutPortSampleTime=0.01
  S-Function : S-Function  FunctionName=s_TD  SFunctionDeploymentMode=off  EnableBusSupport=off
  S-Function4 : S-Function  FunctionName=s_HESO  SFunctionDeploymentMode=off  EnableBusSupport=off
  Scope3 : Scope
  Sum : Sum  Inputs=|+-
  Sum1 : Sum  Inputs=|+-
  Sum2 : Sum  Inputs=++|
  Sum3 : Sum  Inputs=|++
  Terminator : Terminator
  Terminator1 : Terminator
  g : Constant  Value=-9.788
  x : Demux  Outputs=3
  a_t : Outport
  wires:
  Gain1/1 -> Add/2
  Mux/1 -> S-Function4/1
  States/1 -> Bus Selector1/1
  ESO/1 -> Sum/2
  Gain3/1 -> Sum2/2
  ESO/3 -> Sum3/1
  <throttle_cmd>/1 -> RT/1
  ESO/2 -> Sum1/2
  Bus Selector1/1 -> x/1  "<X_ned>"
  RT/1 -> S-Function/1
  S-Function4/1 -> ESO/1
  Sum1/1 -> Gain1/1
  Gain/1 -> Add/1
  RT1/1 -> Demux/1
  Demux/2 -> Sum1/1
  Gain2/1 -> Add/3, Scope3/1
  S-Function/1 -> RT1/1
  Sum/1 -> Gain/1
  Demux/1 -> Sum/1
  x/3 -> Mux/1
  x/2 -> Terminator/1
  x/1 -> Terminator1/1
  Add/1 -> Add2/2, Gain3/1  "a"
  Sum2/1 -> Mux/2
  Sum3/1 -> Gain2/1
  Add2/1 -> a_t/1
  g/1 -> Add2/1

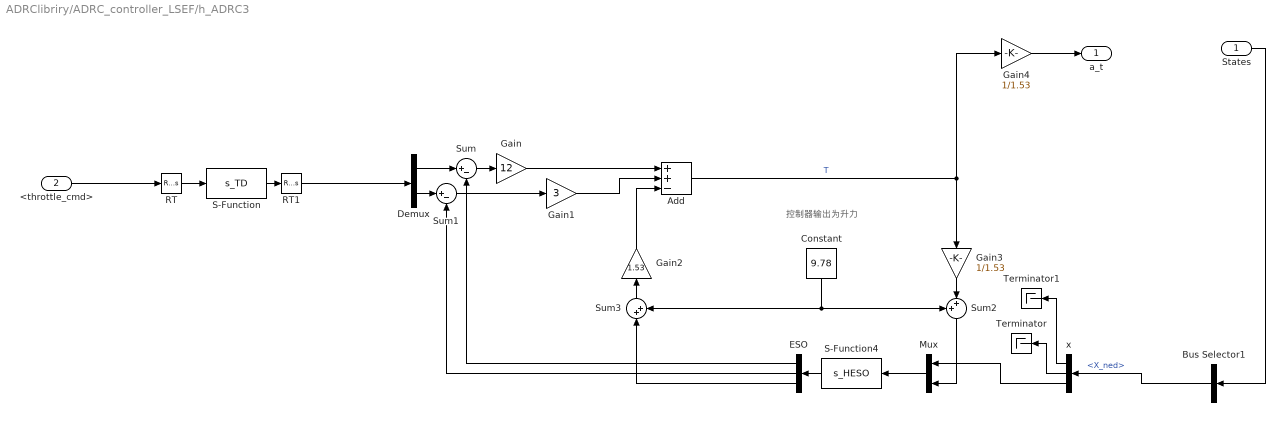
== system ADRClibriry/ADRC_controller_LSEF/h_ADRC3 ==
  note: 控制器输出为升力
  States : Inport  OutDataTypeStr=Bus: StatesBus
  <throttle_cmd> : Inport  Port=2
  Add : Sum  Inputs=++-
  Bus Selector1 : BusSelector  OutputSignals=X_ned
  Constant : Constant  Value=9.78
  Demux : Demux  Outputs=2
  ESO : Demux  Outputs=3
  Gain : Gain  Gain=12
  Gain1 : Gain  Gain=3
  Gain2 : Gain  Gain=1.53
  Gain3 : Gain  Gain=1/1.53
  Gain4 : Gain  Gain=1/1.53
  Mux : Mux  Inputs=2
  RT : RateTransition  OutPortSampleTime=0.05
  RT1 : RateTransition  OutPortSampleTime=0.01
  S-Function : S-Function  FunctionName=s_TD  SFunctionDeploymentMode=off  EnableBusSupport=off
  S-Function4 : S-Function  FunctionName=s_HESO  SFunctionDeploymentMode=off  EnableBusSupport=off
  Sum : Sum  Inputs=|+-
  Sum1 : Sum  Inputs=|+-
  Sum2 : Sum  Inputs=++|
  Sum3 : Sum  Inputs=|++
  Terminator : Terminator
  Terminator1 : Terminator
  x : Demux  Outputs=3
  a_t : Outport
  wires:
  Gain1/1 -> Add/2
  Mux/1 -> S-Function4/1
  States/1 -> Bus Selector1/1
  ESO/1 -> Sum/2
  Gain3/1 -> Sum2/2
  ESO/3 -> Sum3/1
  <throttle_cmd>/1 -> RT/1
  ESO/2 -> Sum1/2
  Bus Selector1/1 -> x/1  "<X_ned>"
  RT/1 -> S-Function/1
  S-Function4/1 -> ESO/1
  Sum1/1 -> Gain1/1
  Gain/1 -> Add/1
  RT1/1 -> Demux/1
  Demux/2 -> Sum1/1
  Gain2/1 -> Add/3
  S-Function/1 -> RT1/1
  Sum/1 -> Gain/1
  Demux/1 -> Sum/1
  x/3 -> Mux/1
  x/2 -> Terminator/1
  x/1 -> Terminator1/1
  Add/1 -> Gain4/1, Gain3/1  "T"
  Sum2/1 -> Mux/2
  Sum3/1 -> Gain2/1
  Constant/1 -> Sum3/2, Sum2/1
  Gain4/1 -> a_t/1

== system ADRClibriry/ADRC_controller_LSEF/pitch_ADRC ==
  States : Inport  OutDataTypeStr=Bus: StatesBus
  <pitch_cmd> : Inport  Port=2
  Add1 : Sum  Inputs=++-
  Bus Selector1 : BusSelector  OutputSignals=Euler
  Demux : Demux  Outputs=2
  ESO : Demux  Outputs=3
  Gain : Gain  Gain=3
  Gain1 : Gain
  Gain4 : Gain  Gain=0.025504
  Gain5 : Gain  Gain=39.2418
  Mux : Mux  Inputs=2
  RT : RateTransition  OutPortSampleTime=0.05
  RT1 : RateTransition  OutPortSampleTime=0.01
  S-Function : S-Function  FunctionName=s_TD  SFunctionDeploymentMode=off  EnableBusSupport=off
  S-Function4 : S-Function  FunctionName=s_ESO  SFunctionDeploymentMode=off  EnableBusSupport=off
  Sum : Sum  Inputs=|+-
  Sum1 : Sum  Inputs=|+-
  Terminator : Terminator
  Terminator1 : Terminator
  angle : Demux  Outputs=3
  u_q : Outport
  wires:
  Gain1/1 -> Add1/2
  Mux/1 -> S-Function4/1
  States/1 -> Bus Selector1/1
  Gain5/1 -> Mux/2
  ESO/3 -> Gain4/1
  Bus Selector1/1 -> angle/1  "<Euler>"
  RT/1 -> S-Function/1
  S-Function4/1 -> ESO/1
  Add1/1 -> Gain5/1, u_q/1
  Sum1/1 -> Gain1/1
  Gain/1 -> Add1/1
  RT1/1 -> Demux/1
  Demux/2 -> Sum1/1
  Gain4/1 -> Add1/3
  S-Function/1 -> RT1/1
  Sum/1 -> Gain/1
  angle/3 -> Terminator1/1
  angle/2 -> Mux/1
  ESO/2 -> Sum1/2
  ESO/1 -> Sum/2
  Demux/1 -> Sum/1
  <pitch_cmd>/1 -> RT/1
  angle/1 -> Terminator/1

== system ADRClibriry/ADRC_controller_LSEF/roll_ADRC ==
  States : Inport  OutDataTypeStr=Bus: StatesBus
  <roll_cmd> : Inport  Port=2
  Add : Sum  Inputs=++-
  Bus Selector1 : BusSelector  OutputSignals=Euler
  ESO : Demux  Outputs=3
  Gain : Gain  Gain=3
  Gain1 : Gain
  Gain2 : Gain  Gain=0.025504
  Gain3 : Gain  Gain=39.2418
  Mux : Mux  Inputs=2
  RT : RateTransition  OutPortSampleTime=0.05
  RT1 : RateTransition  OutPortSampleTime=0.01
  S-Function : S-Function  FunctionName=s_TD  SFunctionDeploymentMode=off  EnableBusSupport=off
  S-Function4 : S-Function  FunctionName=s_ESO  SFunctionDeploymentMode=off  EnableBusSupport=off
  Scope : Scope  NumInputPorts=2
  Scope1 : Scope
  Scope2 : Scope  NumInputPorts=2
  Sum : Sum  Inputs=|+-
  Sum1 : Sum  Inputs=|+-
  TD : Demux  Outputs=2
  Terminator : Terminator
  Terminator1 : Terminator
  angle : Demux  Outputs=3
  "u_p " : Outport
  wires:
  Gain1/1 -> Add/2
  Mux/1 -> S-Function4/1
  States/1 -> Bus Selector1/1
  ESO/1 -> Scope2/1, Sum/2
  Gain3/1 -> Mux/2
  ESO/3 -> Gain2/1
  <roll_cmd>/1 -> Scope/1, RT/1
  angle/1 -> Scope2/2, Mux/1
  ESO/2 -> Sum1/2
  Bus Selector1/1 -> angle/1  "<Euler>"
  RT/1 -> S-Function/1
  S-Function4/1 -> ESO/1
  Add/1 -> "u_p "/1, Gain3/1
  Sum1/1 -> Gain1/1
  Gain/1 -> Add/1
  RT1/1 -> TD/1
  TD/2 -> Scope1/1, Sum1/1
  Gain2/1 -> Add/3
  S-Function/1 -> RT1/1
  Sum/1 -> Gain/1
  TD/1 -> Scope/2, Sum/1
  angle/3 -> Terminator1/1
  angle/2 -> Terminator/1

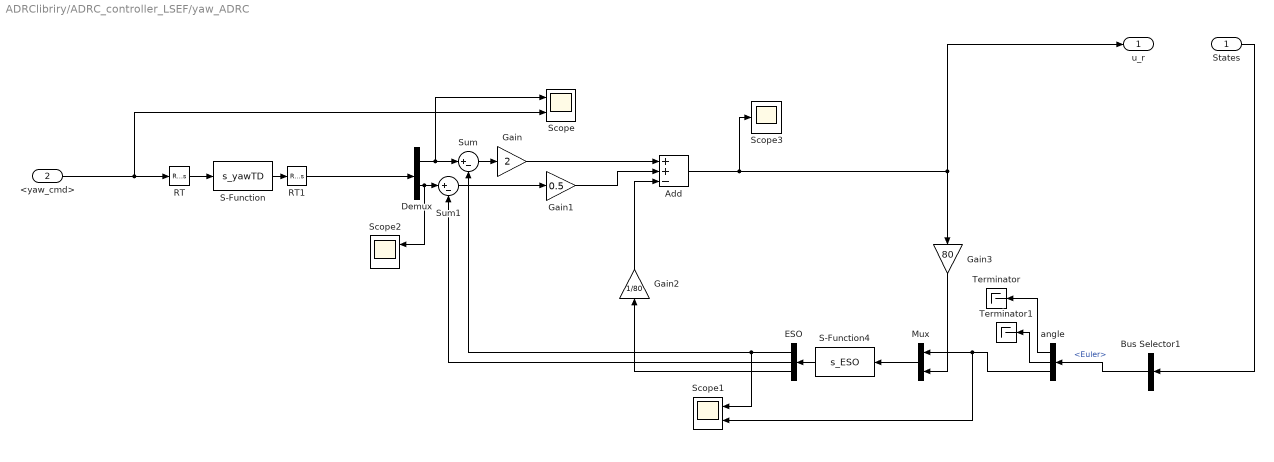
== system ADRClibriry/ADRC_controller_LSEF/yaw_ADRC ==
  States : Inport  OutDataTypeStr=Bus: StatesBus
  <yaw_cmd> : Inport  Port=2
  Add : Sum  Inputs=++-
  Bus Selector1 : BusSelector  OutputSignals=Euler
  Demux : Demux  Outputs=2
  ESO : Demux  Outputs=3
  Gain : Gain  Gain=2
  Gain1 : Gain  Gain=0.5
  Gain2 : Gain  Gain=1/80
  Gain3 : Gain  Gain=80
  Mux : Mux  Inputs=2
  RT : RateTransition
  RT1 : RateTransition
  S-Function : S-Function  FunctionName=s_yawTD  SFunctionDeploymentMode=off  EnableBusSupport=off
  S-Function4 : S-Function  FunctionName=s_ESO  SFunctionDeploymentMode=off  EnableBusSupport=off
  Scope : Scope  NumInputPorts=2
  Scope1 : Scope  NumInputPorts=2
  Scope2 : Scope  NumInputPorts=2
  Scope3 : Scope
  Sum : Sum  Inputs=|+-
  Sum1 : Sum  Inputs=|+-
  Terminator : Terminator
  Terminator1 : Terminator
  angle : Demux  Outputs=3
  u_r : Outport
  wires:
  Gain1/1 -> Add/2
  Mux/1 -> S-Function4/1
  States/1 -> Bus Selector1/1
  ESO/1 -> Scope1/1, Sum/2
  Gain3/1 -> Mux/2
  ESO/3 -> Gain2/1
  <yaw_cmd>/1 -> Scope/2, RT/1
  ESO/2 -> Sum1/2
  Bus Selector1/1 -> angle/1  "<Euler>"
  RT/1 -> S-Function/1
  S-Function4/1 -> ESO/1
  Add/1 -> Scope3/1, u_r/1, Gain3/1
  Sum1/1 -> Gain1/1
  Gain/1 -> Add/1
  RT1/1 -> Demux/1
  Demux/2 -> Scope2/1, Sum1/1
  Gain2/1 -> Add/3
  S-Function/1 -> RT1/1
  Sum/1 -> Gain/1
  Demux/1 -> Scope/1, Sum/1
  angle/3 -> Scope1/2, Mux/1
  angle/2 -> Terminator1/1
  angle/1 -> Terminator/1

== system ADRClibriry/ADRC_controller_NLSEF/Subsystem ==
  In1 : Inport
  In2 : Inport  Port=2
  In3 : Inport  Port=3
  Divide : Product  Inputs=*/
  Gain : Gain  Gain=-1225^2/9.788
  Product : Product
  Saturation1 : Saturate  UpperLimit=1  LowerLimit=0.5
  Sqrt : Sqrt  SaturateOnIntegerOverflow=on
  Trigonometric Function : Trigonometry  Operator=cos
  Trigonometric Function1 : Trigonometry  Operator=cos
  speed : Outport
  wires:
  Saturation1/1 -> Divide/2
  Trigonometric Function/1 -> Product/1
  In3/1 -> Divide/1
  Trigonometric Function1/1 -> Product/2
  In2/1 -> Trigonometric Function/1
  Product/1 -> Saturation1/1
  In1/1 -> Trigonometric Function1/1
  Divide/1 -> Gain/1
  Gain/1 -> Sqrt/1
  Sqrt/1 -> speed/1

== system ADRClibriry/ADRC_controller_NLSEF/Subsystem2 ==
  u_1 : Inport
  u_2 : Inport  Port=2
  u_3 : Inport  Port=3
  Demux3 : Demux
  MATLAB Function : MATLAB Function  TreatAsAtomicUnit=on
  Mux : Mux  Inputs=3
  Saturation{1..4} (4 alike) : Saturate  UpperLimit=0.3491  LowerLimit=-0.3491
  c1 : Outport
  c2 : Outport  Port=2
  c3 : Outport  Port=3
  c4 : Outport  Port=4
  wires:
  Demux3/4 -> Saturation4/1
  Saturation3/1 -> c3/1  "c3"
  u_3/1 -> Mux/3
  u_1/1 -> Mux/1
  Saturation1/1 -> c1/1  "c1"
  Demux3/1 -> Saturation1/1
  Saturation4/1 -> c4/1  "c4"
  Demux3/2 -> Saturation2/1
  u_2/1 -> Mux/2
  Saturation2/1 -> c2/1  "c2"
  Demux3/3 -> Saturation3/1
  Mux/1 -> MATLAB Function/1(u)
  MATLAB Function/1(y) -> Demux3/1

== system ADRClibriry/ADRC_controller_NLSEF/Subsystem3 ==
  u_p : Inport
  u_q : Inport  Port=2
  u_r : Inport  Port=3
  p : Inport  Port=4
  q : Inport  Port=5
  speed : Inport  Port=6
  Add1 : Sum
  Add2 : Sum  Inputs=+-
  Add3 : Sum  Inputs=+-
  Constant1 : Constant  Value=0.000029
  Constant2 : Constant  Value=0.04238
  Product{,1..3} (4 alike) : Product
  u_1 : Outport
  u_2 : Outport  Port=2
  u_3 : Outport  Port=3
  wires:
  Add3/1 -> u_3/1
  Add1/1 -> u_1/1
  Constant1/1 -> Product1/1, Product/2
  q/1 -> Product/1
  Product1/1 -> Product2/1
  Constant2/1 -> Add3/2
  u_p/1 -> Add1/2
  p/1 -> Product1/2
  Add2/1 -> u_2/1
  Product3/1 -> Add1/1
  speed/1 -> Product3/2, Product2/2
  Product/1 -> Product3/1
  Product2/1 -> Add2/2
  u_q/1 -> Add2/1
  u_r/1 -> Add3/1

== system ADRClibriry/ADRC_controller_NLSEF/h_ADRC ==
  note: 控制器输出为升力提供的加速度
  States : Inport  OutDataTypeStr=Bus: StatesBus
  <throttle_cmd> : Inport  Port=2
  Add : Sum  Inputs=+-
  Bus Selector1 : BusSelector  OutputSignals=X_ned
  Constant : Constant  Value=9.78
  Demux : Demux  Outputs=2
  ESO : Demux  Outputs=3
  Gain2 : Gain
  Gain3 : Gain
  MATLAB Function : MATLAB Function  TreatAsAtomicUnit=on
  Mux : Mux  Inputs=2
  RT : RateTransition  OutPortSampleTime=0.05
  RT1 : RateTransition  OutPortSampleTime=0.01
  S-Function : S-Function  FunctionName=s_TD  SFunctionDeploymentMode=off  EnableBusSupport=off
  S-Function4 : S-Function  FunctionName=s_ESO  SFunctionDeploymentMode=off  EnableBusSupport=off
  Scope3 : Scope
  Sum2 : Sum  Inputs=++|
  Sum3 : Sum  Inputs=|++
  Terminator : Terminator
  Terminator1 : Terminator
  x : Demux  Outputs=3
  a_t : Outport
  wires:
  Mux/1 -> S-Function4/1
  States/1 -> Bus Selector1/1
  ESO/1 -> MATLAB Function/3(x1)
  Gain3/1 -> Sum2/2
  ESO/3 -> Sum3/1
  <throttle_cmd>/1 -> RT/1
  ESO/2 -> MATLAB Function/4(x2)
  Bus Selector1/1 -> x/1  "<X_ned>"
  RT/1 -> S-Function/1
  S-Function4/1 -> ESO/1
  RT1/1 -> Demux/1
  Demux/2 -> MATLAB Function/2(x2_d)
  Gain2/1 -> Add/2, Scope3/1
  S-Function/1 -> RT1/1
  Demux/1 -> MATLAB Function/1(x1_d)
  x/3 -> Mux/1
  x/2 -> Terminator/1
  x/1 -> Terminator1/1
  Add/1 -> a_t/1, Gain3/1  "a_t"
  Sum2/1 -> Mux/2
  Sum3/1 -> Gain2/1
  Constant/1 -> Sum3/2, Sum2/1
  MATLAB Function/1(y) -> Add/1

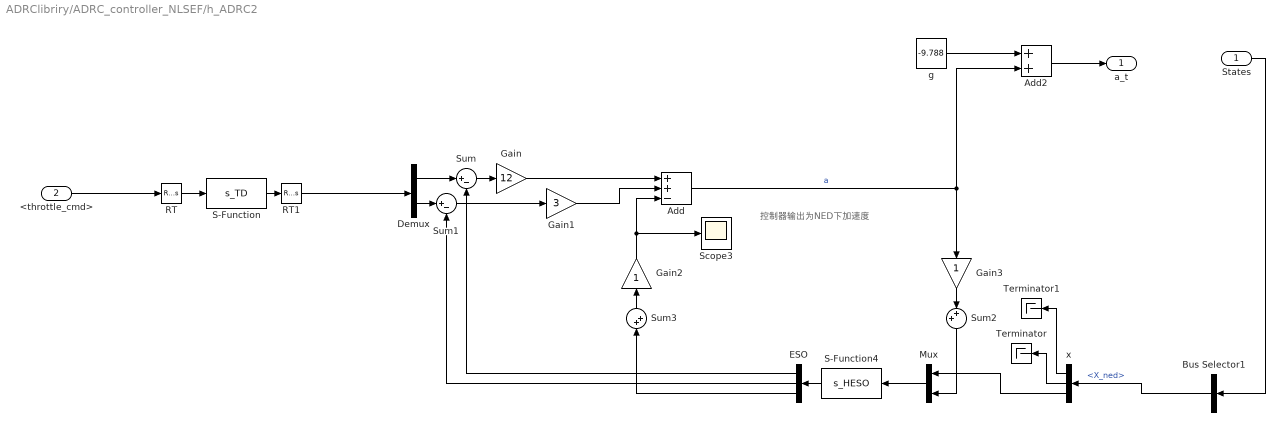
== system ADRClibriry/ADRC_controller_NLSEF/h_ADRC2 ==
  note: 控制器输出为NED下加速度
  States : Inport  OutDataTypeStr=Bus: StatesBus
  <throttle_cmd> : Inport  Port=2
  Add : Sum  Inputs=++-
  Add2 : Sum
  Bus Selector1 : BusSelector  OutputSignals=X_ned
  Demux : Demux  Outputs=2
  ESO : Demux  Outputs=3
  Gain : Gain  Gain=12
  Gain1 : Gain  Gain=3
  Gain2 : Gain
  Gain3 : Gain
  Mux : Mux  Inputs=2
  RT : RateTransition  OutPortSampleTime=0.05
  RT1 : RateTransition  OutPortSampleTime=0.01
  S-Function : S-Function  FunctionName=s_TD  SFunctionDeploymentMode=off  EnableBusSupport=off
  S-Function4 : S-Function  FunctionName=s_HESO  SFunctionDeploymentMode=off  EnableBusSupport=off
  Scope3 : Scope
  Sum : Sum  Inputs=|+-
  Sum1 : Sum  Inputs=|+-
  Sum2 : Sum  Inputs=++|
  Sum3 : Sum  Inputs=|++
  Terminator : Terminator
  Terminator1 : Terminator
  g : Constant  Value=-9.788
  x : Demux  Outputs=3
  a_t : Outport
  wires:
  Gain1/1 -> Add/2
  Mux/1 -> S-Function4/1
  States/1 -> Bus Selector1/1
  ESO/1 -> Sum/2
  Gain3/1 -> Sum2/2
  ESO/3 -> Sum3/1
  <throttle_cmd>/1 -> RT/1
  ESO/2 -> Sum1/2
  Bus Selector1/1 -> x/1  "<X_ned>"
  RT/1 -> S-Function/1
  S-Function4/1 -> ESO/1
  Sum1/1 -> Gain1/1
  Gain/1 -> Add/1
  RT1/1 -> Demux/1
  Demux/2 -> Sum1/1
  Gain2/1 -> Add/3, Scope3/1
  S-Function/1 -> RT1/1
  Sum/1 -> Gain/1
  Demux/1 -> Sum/1
  x/3 -> Mux/1
  x/2 -> Terminator/1
  x/1 -> Terminator1/1
  Add/1 -> Add2/2, Gain3/1  "a"
  Sum2/1 -> Mux/2
  Sum3/1 -> Gain2/1
  Add2/1 -> a_t/1
  g/1 -> Add2/1

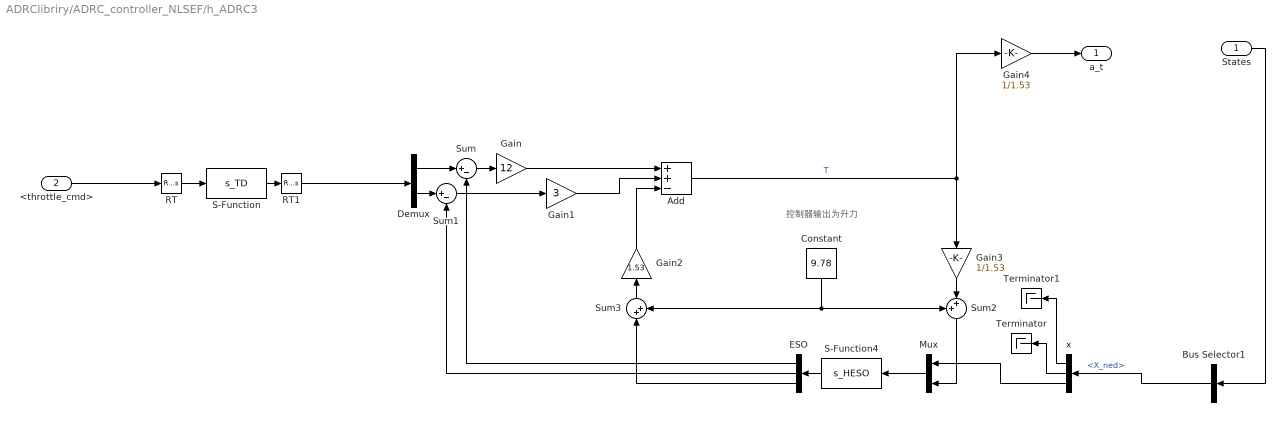
== system ADRClibriry/ADRC_controller_NLSEF/h_ADRC3 ==
  note: 控制器输出为升力
  States : Inport  OutDataTypeStr=Bus: StatesBus
  <throttle_cmd> : Inport  Port=2
  Add : Sum  Inputs=++-
  Bus Selector1 : BusSelector  OutputSignals=X_ned
  Constant : Constant  Value=9.78
  Demux : Demux  Outputs=2
  ESO : Demux  Outputs=3
  Gain : Gain  Gain=12
  Gain1 : Gain  Gain=3
  Gain2 : Gain  Gain=1.53
  Gain3 : Gain  Gain=1/1.53
  Gain4 : Gain  Gain=1/1.53
  Mux : Mux  Inputs=2
  RT : RateTransition  OutPortSampleTime=0.05
  RT1 : RateTransition  OutPortSampleTime=0.01
  S-Function : S-Function  FunctionName=s_TD  SFunctionDeploymentMode=off  EnableBusSupport=off
  S-Function4 : S-Function  FunctionName=s_HESO  SFunctionDeploymentMode=off  EnableBusSupport=off
  Sum : Sum  Inputs=|+-
  Sum1 : Sum  Inputs=|+-
  Sum2 : Sum  Inputs=++|
  Sum3 : Sum  Inputs=|++
  Terminator : Terminator
  Terminator1 : Terminator
  x : Demux  Outputs=3
  a_t : Outport
  wires:
  Gain1/1 -> Add/2
  Mux/1 -> S-Function4/1
  States/1 -> Bus Selector1/1
  ESO/1 -> Sum/2
  Gain3/1 -> Sum2/2
  ESO/3 -> Sum3/1
  <throttle_cmd>/1 -> RT/1
  ESO/2 -> Sum1/2
  Bus Selector1/1 -> x/1  "<X_ned>"
  RT/1 -> S-Function/1
  S-Function4/1 -> ESO/1
  Sum1/1 -> Gain1/1
  Gain/1 -> Add/1
  RT1/1 -> Demux/1
  Demux/2 -> Sum1/1
  Gain2/1 -> Add/3
  S-Function/1 -> RT1/1
  Sum/1 -> Gain/1
  Demux/1 -> Sum/1
  x/3 -> Mux/1
  x/2 -> Terminator/1
  x/1 -> Terminator1/1
  Add/1 -> Gain4/1, Gain3/1  "T"
  Sum2/1 -> Mux/2
  Sum3/1 -> Gain2/1
  Constant/1 -> Sum3/2, Sum2/1
  Gain4/1 -> a_t/1

== system ADRClibriry/ADRC_controller_NLSEF/pitch_ADRC ==
  States : Inport  OutDataTypeStr=Bus: StatesBus
  <pitch_cmd> : Inport  Port=2
  Add1 : Sum  Inputs=+-
  Bus Selector1 : BusSelector  OutputSignals=Euler
  Demux : Demux  Outputs=2
  ESO : Demux  Outputs=3
  Gain4 : Gain  Gain=0.025504
  Gain5 : Gain  Gain=39.2418
  MATLAB Function : MATLAB Function  TreatAsAtomicUnit=on
  Mux : Mux  Inputs=2
  RT : RateTransition  OutPortSampleTime=0.05
  RT1 : RateTransition  OutPortSampleTime=0.01
  S-Function : S-Function  FunctionName=s_TD  SFunctionDeploymentMode=off  EnableBusSupport=off
  S-Function4 : S-Function  FunctionName=s_ESO  SFunctionDeploymentMode=off  EnableBusSupport=off
  Scope4 : Scope  NumInputPorts=2
  Sine Wave : Sin  Amplitude=0.2  Frequency=2*pi*1  SampleTime=0.01
  Terminator : Terminator
  Terminator1 : Terminator
  angle : Demux  Outputs=3
  u_q : Outport
  wires:
  Mux/1 -> S-Function4/1
  States/1 -> Bus Selector1/1
  Gain5/1 -> Mux/2
  ESO/3 -> Gain4/1
  Bus Selector1/1 -> angle/1  "<Euler>"
  RT/1 -> S-Function/1
  S-Function4/1 -> ESO/1
  Add1/1 -> u_q/1, Gain5/1
  RT1/1 -> Demux/1
  Demux/2 -> MATLAB Function/2(x2_d)
  Gain4/1 -> Add1/2
  S-Function/1 -> RT1/1
  angle/3 -> Terminator1/1
  angle/2 -> Mux/1
  ESO/2 -> MATLAB Function/4(x2)
  Demux/1 -> MATLAB Function/1(x1_d)
  <pitch_cmd>/1 -> RT/1
  angle/1 -> Terminator/1
  MATLAB Function/1(y) -> Add1/1
  ESO/1 -> MATLAB Function/3(x1)
  Sine Wave/1 -> Scope4/1

== system ADRClibriry/ADRC_controller_NLSEF/roll_ADRC ==
  States : Inport  OutDataTypeStr=Bus: StatesBus
  <roll_cmd> : Inport  Port=2
  Add : Sum  Inputs=+-
  Bus Selector1 : BusSelector  OutputSignals=Euler
  ESO : Demux  Outputs=3
  Gain2 : Gain  Gain=0.025504
  Gain3 : Gain  Gain=39.2418
  MATLAB Function : MATLAB Function  TreatAsAtomicUnit=on
  Mux : Mux  Inputs=2
  RT : RateTransition  OutPortSampleTime=0.05
  RT1 : RateTransition  OutPortSampleTime=0.01
  S-Function : S-Function  FunctionName=s_TD  SFunctionDeploymentMode=off  EnableBusSupport=off
  S-Function4 : S-Function  FunctionName=s_ESO  SFunctionDeploymentMode=off  EnableBusSupport=off
  Scope : Scope  NumInputPorts=2
  Scope1 : Scope
  Scope2 : Scope  NumInputPorts=2
  Scope4 : Scope  NumInputPorts=2
  Sine Wave : Sin  Amplitude=0.2  Frequency=2*pi*1  Phase=2*pi*1.5  SampleTime=0.01
  TD : Demux  Outputs=2
  Terminator : Terminator
  Terminator1 : Terminator
  angle : Demux  Outputs=3
  "u_p " : Outport
  wires:
  Mux/1 -> S-Function4/1
  States/1 -> Bus Selector1/1
  Gain3/1 -> Mux/2
  ESO/3 -> Gain2/1
  <roll_cmd>/1 -> RT/1, Scope/1
  angle/1 -> Scope2/2, Mux/1
  Bus Selector1/1 -> angle/1  "<Euler>"
  RT/1 -> S-Function/1
  S-Function4/1 -> ESO/1
  Add/1 -> "u_p "/1, Gain3/1
  RT1/1 -> TD/1
  TD/2 -> MATLAB Function/2(x2_d), Scope1/1
  Gain2/1 -> Add/2
  S-Function/1 -> RT1/1
  TD/1 -> MATLAB Function/1(x1_d), Scope/2
  angle/3 -> Terminator1/1
  angle/2 -> Terminator/1
  ESO/2 -> MATLAB Function/4(x2)
  MATLAB Function/1(y) -> Add/1
  Sine Wave/1 -> Scope4/1
  ESO/1 -> MATLAB Function/3(x1), Scope2/1
